simulink model "unipolar"  (R2016b)
settings: Solver=VariableStepDiscrete  StartTime=0.0  StopTime=0.2  RelTol=1e-3
libraries: powerlib x10, simulink x2
settings Model: Creator=Youssef  LastModifiedBy=Youssef

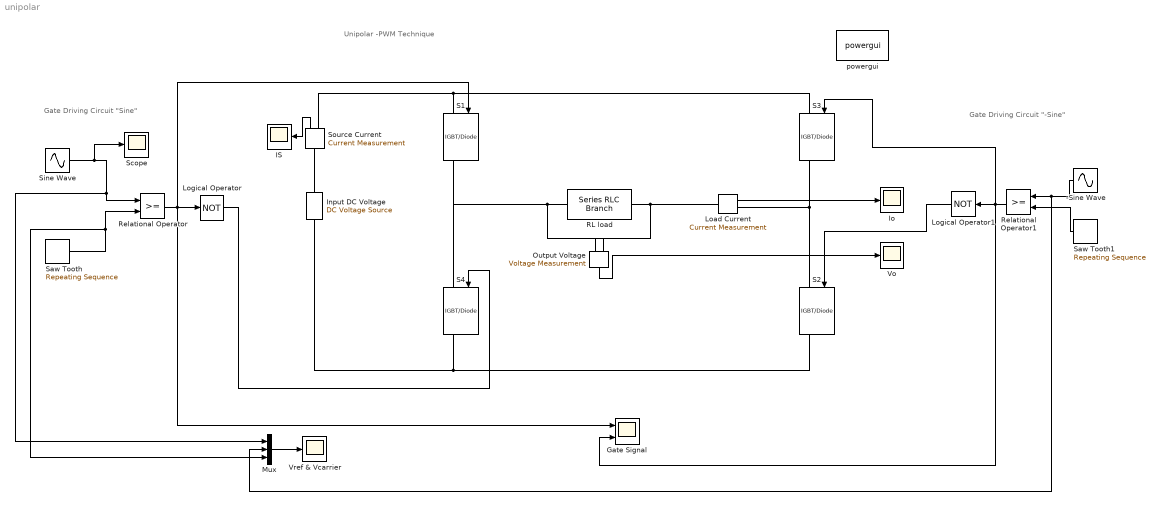
== system unipolar ==
  note: Unipolar -PWM Technique
  note: Gate Driving Circuit "Sine"
  note: Gate Driving Circuit
      | "-Sine"
  -Sine Wave : Sin  Amplitude=0.778  Frequency=2*pi*50  Phase=pi  SampleTime=0
  Gate Signal : Scope  NumInputPorts=2
  IS : Scope
  "Input DC Voltage " : powerlib/Electrical Sources/DC Voltage Source  Amplitude=20  Measurements=None
  Io : Scope
  Load Current : powerlib/Measurements/Current Measurement  PhasorSimulation=off  OutputType=Complex  PSBequivalent=0
  Logical Operator : Logic  Operator=NOT  AllPortsSameDT=off  OutDataTypeStr=boolean
  Logical Operator1 : Logic  Operator=NOT  AllPortsSameDT=off  OutDataTypeStr=boolean
  Mux : Mux  Inputs=3
  "Output Voltage " : powerlib/Measurements/Voltage Measurement  PhasorSimulation=off  OutputType=Complex  PSBequivalent=0
  RL load : powerlib/Elements/Series RLC Branch  LConnTagsString=__new0  RConnTagsString=__new0  BranchType=RL  Resistance=34  Inductance=33e-3  SetiL0=off  InitialCurrent=0  Capacitance=1e-6  Setx0=off  InitialVoltage=0  Measurements=None
  Relational Operator : RelationalOperator  OutDataTypeStr=boolean  RndMeth=Simplest
  Relational Operator1 : RelationalOperator  OutDataTypeStr=boolean  RndMeth=Simplest
  "S1 " : powerlib/Power Electronics/IGBT//Diode  Ron=1e-3  Rs=1e5  Cs=inf  Measurements=on
  "S2 " : powerlib/Power Electronics/IGBT//Diode  Ron=1e-3  Rs=1e5  Cs=inf  Measurements=on
  "S3 " : powerlib/Power Electronics/IGBT//Diode  Ron=1e-3  Rs=1e5  Cs=inf  Measurements=on
  "S4 " : powerlib/Power Electronics/IGBT//Diode  Ron=1e-3  Rs=1e5  Cs=inf  Measurements=on
  Saw Tooth : simulink/Sources/Repeating Sequence  rep_seq_t=[0 (1/10000)/4 (1/10000)/2 (3/10000)/4 (1/10000)]  rep_seq_y=[0 1 0 -1 0]
  Saw Tooth1 : simulink/Sources/Repeating Sequence  rep_seq_t=[0 (1/10000)/4 (1/10000)/2 (3/10000)/4 (1/10000)]  rep_seq_y=[0 1 0 -1 0]
  Scope : Scope
  Sine Wave : Sin  Amplitude=0.778  Frequency=2*pi*50  SampleTime=0
  "Source Current " : powerlib/Measurements/Current Measurement  PhasorSimulation=off  OutputType=Complex  PSBequivalent=0
  Vo : Scope
  Vref & Vcarrier : Scope
  powergui : powerlib/powergui  Priority=1  SimulationMode=Discrete  SolverType=Tustin/Backward Euler (TBE)  SampleTime=1e-6  frequency=60  SPID=off  DisableSnubberDevices=off  DisableRonSwitches=off  DisableVfSwitches=off  SwTol=0  DisplayEquations=off  Interpol=off  ExternalGateDelay=off  methode=off  Ts=10  FunctionMessages=off  echomessages=off  HookPort=off  EnableUseOfTLC=off  x0status=blocks  frequencyindice=0  Pbase=100e6  ErrMax=1e-4  Iterations=50  UnitsV=kV  UnitsW=MW  buscounter=0  RestoreLinks=warning  ResistiveCurrentMeasurement=off  Frange=[0:2:500]  Ylog=off  Xlog=on  ShowGrid=off  save=off  variable=ZData  structure=Ibipolar  ZoomFFT=off  StartTime=0.08  cycles=2  DisplayStyle=1  fundamental=50  FreqAxis=on  MaxFrequency=12000  frequencyindicesteady=1  RmsSteady=1  display=off
  wires:
  "Output Voltage "/1 -> Vo/1
  Load Current/1 -> Io/1
  Sine Wave/1 -> Scope/1, Mux/1, Relational Operator/1
  Saw Tooth/1 -> Mux/3, Relational Operator/2
  Relational Operator/1 -> "S1 "/1, Logical Operator/1, Gate Signal/1
  Logical Operator/1 -> "S4 "/1
  "Source Current "/1 -> IS/1
  -Sine Wave/1 -> Mux/2, Relational Operator1/1
  Saw Tooth1/1 -> Relational Operator1/2
  Relational Operator1/1 -> Gate Signal/2, Logical Operator1/1, "S3 "/1
  Logical Operator1/1 -> "S2 "/1
  Mux/1 -> Vref & Vcarrier/1
  connections:
  "Input DC Voltage "/RConn1 -- "Source Current "/LConn1
  "Source Current "/RConn1 -- "S3 "/LConn1 -- "S1 "/LConn1
  "S4 "/LConn1 -- "S1 "/RConn1 -- RL load/LConn1 -- "Output Voltage "/LConn2
  Load Current/RConn1 -- "S3 "/RConn1 -- "S2 "/LConn1
  "Input DC Voltage "/LConn1 -- "S4 "/RConn1 -- "S2 "/RConn1
  Load Current/LConn1 -- RL load/RConn1 -- "Output Voltage "/LConn1
